simulink model "model"  (Simulink 7.7)
settings: Solver=ode45  StartTime=0.0  StopTime=10000.0  RelTol=1e-3
libraries: simeventsattributes2 x23, simeventsgenerators1 x10, simeventsrouting1 x7, simeventsserver1 x5, simeventsqueue1 x2, simeventssink1 x1, simulink x1
settings Model: Creator=flp  LastModifiedBy=flp
settings SimEventsCC: propDiagAttribOutput=1  propDiagFcnCallOutput=1  propDiagStatOutput=0

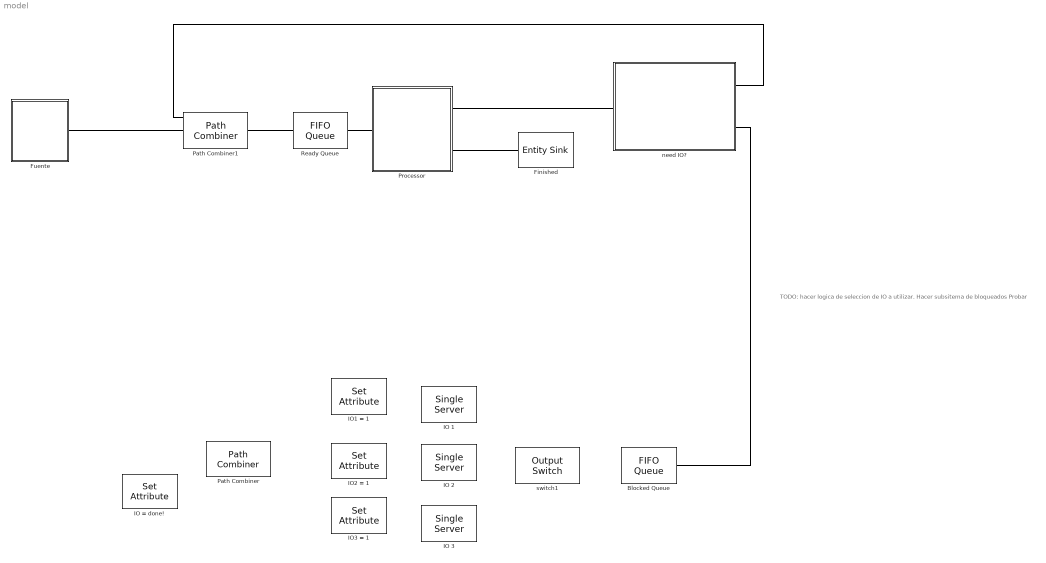
== system model ==
  note: TODO:
      |
      | hacer logica de seleccion de IO a utilizar.
      | Hacer subsitema de bloqueados
      | Probar
  Blocked Queue : simeventsqueue1/FIFO Queue  SystemSampleTime=-1  Capacity=25  EnableTOPort=off  StatNumberDeparted=Off  StatNumberInBlock=Off  StatPendingEntity=Off  StatAverageWait=Off  StatAverageQueueLength=Off  StatNumberTimedout=Off
  Finished : simeventssink1/Entity Sink  SystemSampleTime=-1  AvailableForArrivals=on  StatNumberArrived=Off
  Fuente : Subsystem
  IO 1 : simeventsserver1/Single Server  SystemSampleTime=-1  ServiceTimeFrom=Signal port t  ServiceTime=1  AttributeName=ServiceTime  PriorityServiceCompletion=500  PermitPreemption=off  SortingAttributeName=PriorityAttributeName  SortingDirection=Ascending  WriteToAttribute=off  ResidualAttributeName=ResidualServiceTime  CreateAttribute=on  EnableTOPort=off  StatNumberDeparted=Off  StatNumberInBlock=Off  StatNumberPreempted=Off  StatPendingEntity=Off  StatAverageWait=Off  StatUtilization=Off  StatNumberTimedout=Off
  IO 2 : simeventsserver1/Single Server  SystemSampleTime=-1  ServiceTimeFrom=Signal port t  ServiceTime=1  AttributeName=ServiceTime  PriorityServiceCompletion=500  PermitPreemption=off  SortingAttributeName=PriorityAttributeName  SortingDirection=Ascending  WriteToAttribute=off  ResidualAttributeName=ResidualServiceTime  CreateAttribute=on  EnableTOPort=off  StatNumberDeparted=Off  StatNumberInBlock=Off  StatNumberPreempted=Off  StatPendingEntity=Off  StatAverageWait=Off  StatUtilization=Off  StatNumberTimedout=Off
  IO 3 : simeventsserver1/Single Server  SystemSampleTime=-1  ServiceTimeFrom=Signal port t  ServiceTime=1  AttributeName=ServiceTime  PriorityServiceCompletion=500  PermitPreemption=off  SortingAttributeName=PriorityAttributeName  SortingDirection=Ascending  WriteToAttribute=off  ResidualAttributeName=ResidualServiceTime  CreateAttribute=on  EnableTOPort=off  StatNumberDeparted=Off  StatNumberInBlock=Off  StatNumberPreempted=Off  StatPendingEntity=Off  StatAverageWait=Off  StatUtilization=Off  StatNumberTimedout=Off
  IO = done! : simeventsattributes2/Set Attribute  SystemSampleTime=-1  AttributeFrom=Dialog  AttributeName=Attribute1  AttributeTreatAsVector=1  AttributeValue=1  AttributeCreate=on  StatNumberDeparted=Off  EvaluatedAttributeValue={1}
  IO1 = 1 : simeventsattributes2/Set Attribute  SystemSampleTime=-1  AttributeFrom=Signal port  AttributeName=current_process_time  AttributeTreatAsVector=1  AttributeValue=1  AttributeCreate=on  StatNumberDeparted=Off  EvaluatedAttributeValue={[]}
  IO2 = 1 : simeventsattributes2/Set Attribute  SystemSampleTime=-1  AttributeFrom=Signal port  AttributeName=current_process_time  AttributeTreatAsVector=1  AttributeValue=1  AttributeCreate=on  StatNumberDeparted=Off  EvaluatedAttributeValue={[]}
  IO3 = 1 : simeventsattributes2/Set Attribute  SystemSampleTime=-1  AttributeFrom=Signal port  AttributeName=current_process_time  AttributeTreatAsVector=1  AttributeValue=1  AttributeCreate=on  StatNumberDeparted=Off  EvaluatedAttributeValue={[]}
  Path Combiner : simeventsrouting1/Path Combiner  SystemSampleTime=-1  NumberInputPorts=3  InputPortPrecedence=IN1 port  InitialSeed=45675  SpecifyEventPriority=off  PriorityPathCombinerPortPrecedenceSelection=4100  StatNumberDeparted=Off  StatLastArrivalPort=Off  EvaluatedNumPorts=3
  Path Combiner1 : simeventsrouting1/Path Combiner  SystemSampleTime=-1  NumberInputPorts=3  InputPortPrecedence=IN1 port  InitialSeed=45675  SpecifyEventPriority=off  PriorityPathCombinerPortPrecedenceSelection=4100  StatNumberDeparted=Off  StatLastArrivalPort=Off  EvaluatedNumPorts=3
  Processor : Subsystem
  Ready Queue : simeventsqueue1/FIFO Queue  SystemSampleTime=-1  Capacity=40  EnableTOPort=off  StatNumberDeparted=Off  StatNumberInBlock=Off  StatPendingEntity=Off  StatAverageWait=Off  StatAverageQueueLength=Off  StatNumberTimedout=Off
  need IO? : Subsystem
  switch1 : simeventsrouting1/Output Switch  SystemSampleTime=-1  NumberOutputPorts=3  SwitchingCriterion=From attribute  InitialSeed=34567  AttributeName=Attribute1  InitialConditionsOpt=off  InitialConditions=1  EntityBufferOpt=off  SpecifyEventPriority=off  PriorityOutputSwitchSelectPort=4100  TimeoutPortOpt=off  StatNumberDeparted=Off  StatNumberTimedOut=Off  StatPendingEntity=Off  StatLastDeparturePort=Off  EvaluatedNumPorts=3
  connections:
  Ready Queue/RConn1 -- Processor/LConn1
  Processor/RConn2 -- Finished/LConn1
  Processor/RConn1 -- need IO?/LConn1
  Fuente/RConn1 -- Path Combiner1/LConn2
  need IO?/RConn1 -- Path Combiner1/LConn1
  Path Combiner1/RConn1 -- Ready Queue/LConn1
  need IO?/RConn2 -- Blocked Queue/LConn1

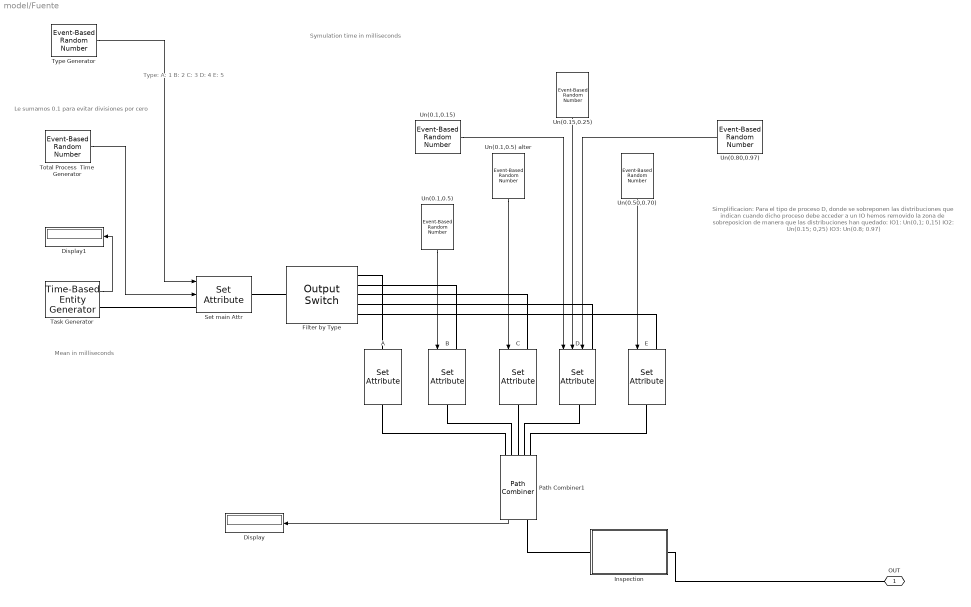
== system model/Fuente ==
  note: Type:
      |
      | A: 1
      | B: 2
      | C: 3
      | D: 4
      | E: 5
  note: Mean in milliseconds
  note: Symulation time in milliseconds
  note: Simplificacion:
      | Para el tipo de proceso D, donde se sobreponen
      | las distribuciones que indican cuando dicho proceso
      | debe acceder a un IO hemos removido la
      | zona de sobreposicion de manera que las
      | distribuciones han quedado:
      |
      | IO1: Un(0,1; 0,15)
      | IO2: Un(0.15; 0,25)
      | IO3: Un(0.8; 0.97)
  note: Le sumamos 0.1 para
      | evitar divisiones por cero
  A : simeventsattributes2/Set Attribute  SystemSampleTime=-1  AttributeFrom=Dialog|Dialog|Dialog  AttributeName=IO1|IO2|IO3  AttributeTreatAsVector=1|1|1  AttributeValue=0|0|0  AttributeCreate=on  StatNumberDeparted=Off  EvaluatedAttributeValue={0;0;0}
  B : simeventsattributes2/Set Attribute  SystemSampleTime=-1  AttributeFrom=Signal port|Dialog|Dialog  AttributeName=IO1|IO2|IO3  AttributeTreatAsVector=1|1|1  AttributeValue=1|0|0  AttributeCreate=on  StatNumberDeparted=Off  EvaluatedAttributeValue={[];0;0}
  C : simeventsattributes2/Set Attribute  SystemSampleTime=-1  AttributeFrom=Dialog|Signal port|Dialog  AttributeName=IO1|IO2|IO3  AttributeTreatAsVector=1|1|1  AttributeValue=0|1|0  AttributeCreate=on  StatNumberDeparted=Off  EvaluatedAttributeValue={0;[];0}
  D : simeventsattributes2/Set Attribute  SystemSampleTime=-1  AttributeFrom=Signal port|Signal port|Signal port  AttributeName=IO1|IO2|IO3  AttributeTreatAsVector=1|1|1  AttributeValue=1|1|1  AttributeCreate=on  StatNumberDeparted=Off  EvaluatedAttributeValue={[];[];[]}
  Display : Display
  Display1 : Display
  E : simeventsattributes2/Set Attribute  SystemSampleTime=-1  AttributeFrom=Dialog|Dialog|Signal port  AttributeName=IO1|IO2|IO3  AttributeTreatAsVector=1|1|1  AttributeValue=0|0|1  AttributeCreate=on  StatNumberDeparted=Off  EvaluatedAttributeValue={0;0;[]}
  Filter by Type : simeventsrouting1/Output Switch  SystemSampleTime=-1  NumberOutputPorts=5  SwitchingCriterion=From attribute  InitialSeed=34567  AttributeName=type  InitialConditionsOpt=off  InitialConditions=1  EntityBufferOpt=off  SpecifyEventPriority=off  PriorityOutputSwitchSelectPort=4100  TimeoutPortOpt=off  StatNumberDeparted=Off  StatNumberTimedOut=Off  StatPendingEntity=Off  StatLastDeparturePort=Off  EvaluatedNumPorts=5
  Inspection : Subsystem
  Path Combiner1 : simeventsrouting1/Path Combiner  SystemSampleTime=-1  NumberInputPorts=5  InputPortPrecedence=IN1 port  InitialSeed=45675  SpecifyEventPriority=off  PriorityPathCombinerPortPrecedenceSelection=4100  StatNumberDeparted=On  StatLastArrivalPort=Off  EvaluatedNumPorts=5
  Set main Attr : simeventsattributes2/Set Attribute  SystemSampleTime=-1  AttributeFrom=Signal port|Signal port|Dialog  AttributeName=type|total_process_time|current_process_time  AttributeTreatAsVector=1|1|1  AttributeValue=1|1|0  AttributeCreate=on  StatNumberDeparted=Off  EvaluatedAttributeValue={[];[];0}
  Task Generator : simeventsgenerators1/Entity Generators/Time-Based Entity Generator  SystemSampleTime=-1  GenerateEntitiesUpon=Intergeneration time from dialog  Distribution=Exponential  Minimum=0  Maximum=1  Mean=212.8  InitialSeed=1234  Period=1  PriorityEntityGeneration=300  GenerateEntityAtSimulationStart=on  ResponseWhenBlocked=Pause generation  ResponseWhenUnblocked=Immediate restart  EntityType=Blank  StatNumberDeparted=On  StatPendingEntity=Off  StatAverageIntergenerationTime=Off
  Total Process  Time Generator : simeventsgenerators1/Signal Generators/Event-Based Random Number  SystemSampleTime=-1  distribution=Gaussian (normal)  meanExp=1  minUnif=1  maxUnif=1  pOneBern=0.25  pSuccessBino=0.5  numTrialBino=1  meanNorm=200  stdNorm=40  minTri=1  maxTri=3  modeTri=2  thresholdLogn=0  scaleLogn=1  shapeLogn=1  pSuccessGeo=0.5  meanPoiss=1  thresholdLogl=0  scaleLogl=1  thresholdGam=0  scaleGam=1  shapeGam=1  minBeta=0  maxBeta=1  shape1Beta=1  shape2Beta=1  minUnid=0  maxUnid=1  numValueUnid=2  thresholdWbl=0  scaleWbl=1  shapeWbl=1  valueVecCont=[0 1]  cdfVecCont=[0 1]  valueVecDisc=[0 1]  probVecDisc=[0.5 0.5]  seed=12357632  IsProcessed=on  isConnected=1
  Type Generator : simeventsgenerators1/Signal Generators/Event-Based Random Number  SystemSampleTime=-1  distribution=Arbitrary discrete  meanExp=1  minUnif=1  maxUnif=1  pOneBern=0.25  pSuccessBino=0.5  numTrialBino=1  meanNorm=0  stdNorm=1  minTri=1  maxTri=3  modeTri=2  thresholdLogn=0  scaleLogn=1  shapeLogn=1  pSuccessGeo=0.5  meanPoiss=1  thresholdLogl=0  scaleLogl=1  thresholdGam=0  scaleGam=1  shapeGam=1  minBeta=0  maxBeta=1  shape1Beta=1  shape2Beta=1  minUnid=0  maxUnid=1  numValueUnid=2  thresholdWbl=0  scaleWbl=1  shapeWbl=1  valueVecCont=[0 1]  cdfVecCont=[0 1]  valueVecDisc=[1 2 3 4 5]  probVecDisc=[0.05 0.15 0.25 0.35 0.20]  seed=5533312  IsProcessed=on  isConnected=1
  Un(0.1,0.15) : simeventsgenerators1/Signal Generators/Event-Based Random Number  SystemSampleTime=-1  distribution=Uniform  meanExp=1  minUnif=0.1  maxUnif=0.15  pOneBern=0.25  pSuccessBino=0.5  numTrialBino=1  meanNorm=200  stdNorm=40  minTri=1  maxTri=3  modeTri=2  thresholdLogn=0  scaleLogn=1  shapeLogn=1  pSuccessGeo=0.5  meanPoiss=1  thresholdLogl=0  scaleLogl=1  thresholdGam=0  scaleGam=1  shapeGam=1  minBeta=0  maxBeta=1  shape1Beta=1  shape2Beta=1  minUnid=0  maxUnid=1  numValueUnid=2  thresholdWbl=0  scaleWbl=1  shapeWbl=1  valueVecCont=[0 1]  cdfVecCont=[0 1]  valueVecDisc=[0 1]  probVecDisc=[0.5 0.5]  seed=19165  IsProcessed=on  isConnected=1
  Un(0.1,0.5) : simeventsgenerators1/Signal Generators/Event-Based Random Number  SystemSampleTime=-1  distribution=Uniform  meanExp=1  minUnif=0.1  maxUnif=0.5  pOneBern=0.25  pSuccessBino=0.5  numTrialBino=1  meanNorm=200  stdNorm=40  minTri=1  maxTri=3  modeTri=2  thresholdLogn=0  scaleLogn=1  shapeLogn=1  pSuccessGeo=0.5  meanPoiss=1  thresholdLogl=0  scaleLogl=1  thresholdGam=0  scaleGam=1  shapeGam=1  minBeta=0  maxBeta=1  shape1Beta=1  shape2Beta=1  minUnid=0  maxUnid=1  numValueUnid=2  thresholdWbl=0  scaleWbl=1  shapeWbl=1  valueVecCont=[0 1]  cdfVecCont=[0 1]  valueVecDisc=[0 1]  probVecDisc=[0.5 0.5]  seed=3786546  IsProcessed=on  isConnected=1
  Un(0.1,0.5) alter : simeventsgenerators1/Signal Generators/Event-Based Random Number  SystemSampleTime=-1  distribution=Uniform  meanExp=1  minUnif=0.1  maxUnif=0.5  pOneBern=0.25  pSuccessBino=0.5  numTrialBino=1  meanNorm=200  stdNorm=40  minTri=1  maxTri=3  modeTri=2  thresholdLogn=0  scaleLogn=1  shapeLogn=1  pSuccessGeo=0.5  meanPoiss=1  thresholdLogl=0  scaleLogl=1  thresholdGam=0  scaleGam=1  shapeGam=1  minBeta=0  maxBeta=1  shape1Beta=1  shape2Beta=1  minUnid=0  maxUnid=1  numValueUnid=2  thresholdWbl=0  scaleWbl=1  shapeWbl=1  valueVecCont=[0 1]  cdfVecCont=[0 1]  valueVecDisc=[0 1]  probVecDisc=[0.5 0.5]  seed=22382  IsProcessed=on  isConnected=1
  Un(0.15,0.25) : simeventsgenerators1/Signal Generators/Event-Based Random Number  SystemSampleTime=-1  distribution=Uniform  meanExp=1  minUnif=0.15  maxUnif=0.25  pOneBern=0.25  pSuccessBino=0.5  numTrialBino=1  meanNorm=200  stdNorm=40  minTri=1  maxTri=3  modeTri=2  thresholdLogn=0  scaleLogn=1  shapeLogn=1  pSuccessGeo=0.5  meanPoiss=1  thresholdLogl=0  scaleLogl=1  thresholdGam=0  scaleGam=1  shapeGam=1  minBeta=0  maxBeta=1  shape1Beta=1  shape2Beta=1  minUnid=0  maxUnid=1  numValueUnid=2  thresholdWbl=0  scaleWbl=1  shapeWbl=1  valueVecCont=[0 1]  cdfVecCont=[0 1]  valueVecDisc=[0 1]  probVecDisc=[0.5 0.5]  seed=25599  IsProcessed=on  isConnected=1
  Un(0.50,0.70) : simeventsgenerators1/Signal Generators/Event-Based Random Number  SystemSampleTime=-1  distribution=Uniform  meanExp=1  minUnif=0.5  maxUnif=0.7  pOneBern=0.25  pSuccessBino=0.5  numTrialBino=1  meanNorm=200  stdNorm=40  minTri=1  maxTri=3  modeTri=2  thresholdLogn=0  scaleLogn=1  shapeLogn=1  pSuccessGeo=0.5  meanPoiss=1  thresholdLogl=0  scaleLogl=1  thresholdGam=0  scaleGam=1  shapeGam=1  minBeta=0  maxBeta=1  shape1Beta=1  shape2Beta=1  minUnid=0  maxUnid=1  numValueUnid=2  thresholdWbl=0  scaleWbl=1  shapeWbl=1  valueVecCont=[0 1]  cdfVecCont=[0 1]  valueVecDisc=[0 1]  probVecDisc=[0.5 0.5]  seed=28816  IsProcessed=on  isConnected=1
  Un(0.80,0.97) : simeventsgenerators1/Signal Generators/Event-Based Random Number  SystemSampleTime=-1  distribution=Uniform  meanExp=1  minUnif=0.8  maxUnif=0.97  pOneBern=0.25  pSuccessBino=0.5  numTrialBino=1  meanNorm=200  stdNorm=40  minTri=1  maxTri=3  modeTri=2  thresholdLogn=0  scaleLogn=1  shapeLogn=1  pSuccessGeo=0.5  meanPoiss=1  thresholdLogl=0  scaleLogl=1  thresholdGam=0  scaleGam=1  shapeGam=1  minBeta=0  maxBeta=1  shape1Beta=1  shape2Beta=1  minUnid=0  maxUnid=1  numValueUnid=2  thresholdWbl=0  scaleWbl=1  shapeWbl=1  valueVecCont=[0 1]  cdfVecCont=[0 1]  valueVecDisc=[0 1]  probVecDisc=[0.5 0.5]  seed=35250  IsProcessed=on  isConnected=1
  OUT : PMIOPort  Port=1  Side=Right
  wires:
  Type Generator/1 -> Set main Attr/1
  Un(0.1,0.5)/1 -> B/1
  Un(0.1,0.5) alter/1 -> C/1
  Un(0.1,0.15)/1 -> D/1
  Un(0.15,0.25)/1 -> D/2
  Un(0.80,0.97)/1 -> D/3
  Un(0.50,0.70)/1 -> E/1
  Task Generator/1 -> Display1/1
  Path Combiner1/1 -> Display/1
  Total Process  Time Generator/1 -> Set main Attr/2
  connections:
  Filter by Type/RConn1 -- A/LConn1
  Filter by Type/RConn2 -- B/LConn1
  Filter by Type/RConn3 -- C/LConn1
  Filter by Type/RConn4 -- D/LConn1
  Filter by Type/RConn5 -- E/LConn1
  Task Generator/RConn1 -- Set main Attr/LConn1
  Set main Attr/RConn1 -- Filter by Type/LConn1
  A/RConn1 -- Path Combiner1/LConn1
  B/RConn1 -- Path Combiner1/LConn2
  C/RConn1 -- Path Combiner1/LConn3
  D/RConn1 -- Path Combiner1/LConn4
  E/RConn1 -- Path Combiner1/LConn5
  Inspection/LConn1 -- Path Combiner1/RConn1
  Inspection/RConn1 -- OUT/RConn1

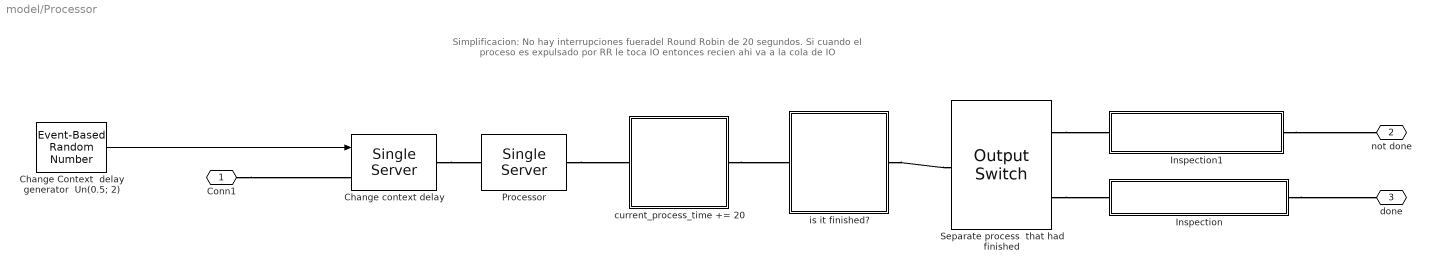
== system model/Processor ==
  note: Simplificacion:
      |
      | No hay interrupciones fueradel
      | Round Robin de 20 segundos.
      | Si cuando el proceso es expulsado por
      | RR le toca IO entonces recien ahi va a
      | la cola de IO
  Change Context  delay generator  Un(0.5; 2) : simeventsgenerators1/Signal Generators/Event-Based Random Number  SystemSampleTime=-1  distribution=Uniform  meanExp=1  minUnif=0.5  maxUnif=2  pOneBern=0.25  pSuccessBino=0.5  numTrialBino=1  meanNorm=0  stdNorm=1  minTri=1  maxTri=3  modeTri=2  thresholdLogn=0  scaleLogn=1  shapeLogn=1  pSuccessGeo=0.5  meanPoiss=1  thresholdLogl=0  scaleLogl=1  thresholdGam=0  scaleGam=1  shapeGam=1  minBeta=0  maxBeta=1  shape1Beta=1  shape2Beta=1  minUnid=0  maxUnid=1  numValueUnid=2  thresholdWbl=0  scaleWbl=1  shapeWbl=1  valueVecCont=[0 1]  cdfVecCont=[0 1]  valueVecDisc=[0 1]  probVecDisc=[0.5 0.5]  seed=55444325  IsProcessed=on  isConnected=1
  Change context delay : simeventsserver1/Single Server  SystemSampleTime=-1  ServiceTimeFrom=Signal port t  ServiceTime=1  AttributeName=ServiceTime  PriorityServiceCompletion=500  PermitPreemption=off  SortingAttributeName=PriorityAttributeName  SortingDirection=Ascending  WriteToAttribute=off  ResidualAttributeName=ResidualServiceTime  CreateAttribute=on  EnableTOPort=off  StatNumberDeparted=Off  StatNumberInBlock=Off  StatNumberPreempted=Off  StatPendingEntity=Off  StatAverageWait=Off  StatUtilization=Off  StatNumberTimedout=Off
  Inspection : Subsystem
  Inspection1 : Subsystem
  Processor : simeventsserver1/Single Server  SystemSampleTime=-1  ServiceTimeFrom=Dialog  ServiceTime=20  AttributeName=ServiceTime  PriorityServiceCompletion=500  PermitPreemption=off  SortingAttributeName=PriorityAttributeName  SortingDirection=Ascending  WriteToAttribute=off  ResidualAttributeName=ResidualServiceTime  CreateAttribute=on  EnableTOPort=off  StatNumberDeparted=Off  StatNumberInBlock=Off  StatNumberPreempted=Off  StatPendingEntity=Off  StatAverageWait=Off  StatUtilization=Off  StatNumberTimedout=Off
  Separate process  that had finished : simeventsrouting1/Output Switch  SystemSampleTime=-1  NumberOutputPorts=2  SwitchingCriterion=From attribute  InitialSeed=34567  AttributeName=done  InitialConditionsOpt=off  InitialConditions=1  EntityBufferOpt=off  SpecifyEventPriority=off  PriorityOutputSwitchSelectPort=4100  TimeoutPortOpt=off  StatNumberDeparted=Off  StatNumberTimedOut=Off  StatPendingEntity=Off  StatLastDeparturePort=Off  EvaluatedNumPorts=2
  current_process_time += 20 : Subsystem
  is it finished? : Subsystem
  Conn1 : PMIOPort  Port=1  Side=Left
  not done : PMIOPort  Port=2  Side=Right
  done : PMIOPort  Port=3  Side=Right
  wires:
  Change Context  delay generator  Un(0.5; 2)/1 -> Change context delay/1
  connections:
  Change context delay/RConn1 -- Processor/LConn1
  Processor/RConn1 -- current_process_time += 20/LConn1
  current_process_time += 20/RConn1 -- is it finished?/LConn1
  Conn1/RConn1 -- Change context delay/LConn1
  is it finished?/RConn1 -- Separate process  that had finished/LConn1
  Separate process  that had finished/RConn1 -- Inspection1/LConn1
  Separate process  that had finished/RConn2 -- Inspection/LConn1
  Inspection/RConn1 -- done/RConn1
  Inspection1/RConn1 -- not done/RConn1

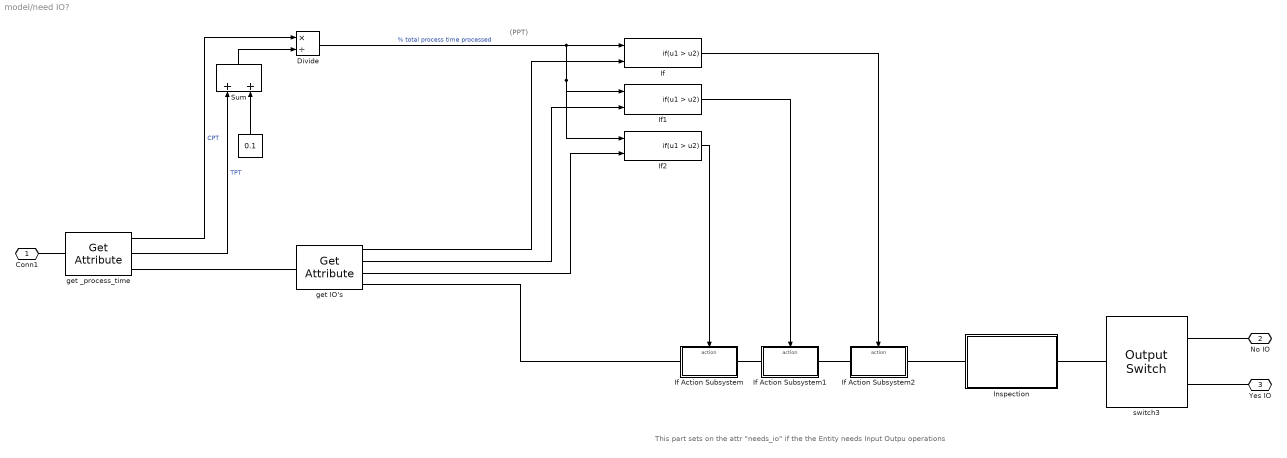
== system model/need IO? ==
  note: (PPT)
  note: This part sets on the attr "needs_io" if the the Entity needs Input Outpu operations
  "   " : Constant  Value=0.1
  Divide : Product  Inputs=*/
  If : If  NumInputs=2  IfExpression=u1 > u2  ShowElse=off
  If Action Subsystem : Subsystem  TreatAsAtomicUnit=on
  If Action Subsystem1 : Subsystem  TreatAsAtomicUnit=on
  If Action Subsystem2 : Subsystem  TreatAsAtomicUnit=on
  If1 : If  NumInputs=2  IfExpression=u1 > u2  ShowElse=off
  If2 : If  NumInputs=2  IfExpression=u1 > u2  ShowElse=off
  Inspection : Subsystem
  Sum : Sum
  get IO's : simeventsattributes2/Get Attribute  SystemSampleTime=-1  AttributeName=IO1|IO2|IO3  AttributeMissing=Error|Error|Error  AttributeDefaultValue=1|1|1  AttributeSendTiming=After entity departure|After entity departure|After entity departure  AttributeTreatAsVector=1|1|1  StatNumberDeparted=Off  EvaluatedDefaultAttributeValue={[];[];[]}
  get _process_time : simeventsattributes2/Get Attribute  SystemSampleTime=-1  AttributeName=current_process_time|total_process_time  AttributeMissing=Error|Error  AttributeDefaultValue=1|1  AttributeSendTiming=After entity departure|After entity departure  AttributeTreatAsVector=1|1  StatNumberDeparted=Off  EvaluatedDefaultAttributeValue={[];[]}
  switch3 : simeventsrouting1/Output Switch  SystemSampleTime=-1  NumberOutputPorts=2  SwitchingCriterion=From attribute  InitialSeed=34567  AttributeName=needs_io  InitialConditionsOpt=off  InitialConditions=1  EntityBufferOpt=off  SpecifyEventPriority=off  PriorityOutputSwitchSelectPort=4100  TimeoutPortOpt=off  StatNumberDeparted=Off  StatNumberTimedOut=Off  StatPendingEntity=Off  StatLastDeparturePort=Off  EvaluatedNumPorts=2
  Conn1 : PMIOPort  Port=1  Side=Left
  No IO : PMIOPort  Port=2  Side=Right
  Yes IO : PMIOPort  Port=3  Side=Right
  wires:
  get _process_time/1 -> Divide/1  "CPT"
  get _process_time/2 -> Sum/1  "TPT"
  Divide/1 -> If/1, If2/1, If1/1  "% total process time processed"
  Sum/1 -> Divide/2
  "   "/1 -> Sum/2
  get IO's/1 -> If/2
  get IO's/2 -> If1/2
  get IO's/3 -> If2/2
  If1/1 -> If Action Subsystem1/Action
  If2/1 -> If Action Subsystem/Action
  If/1 -> If Action Subsystem2/Action
  connections:
  get _process_time/RConn1 -- get IO's/LConn1
  Conn1/RConn1 -- get _process_time/LConn1
  No IO/RConn1 -- switch3/RConn1
  Yes IO/RConn1 -- switch3/RConn2
  If Action Subsystem/RConn1 -- If Action Subsystem1/LConn1
  If Action Subsystem1/RConn1 -- If Action Subsystem2/LConn1
  get IO's/RConn1 -- If Action Subsystem/LConn1
  Inspection/RConn1 -- switch3/LConn1
  If Action Subsystem2/RConn1 -- Inspection/LConn1

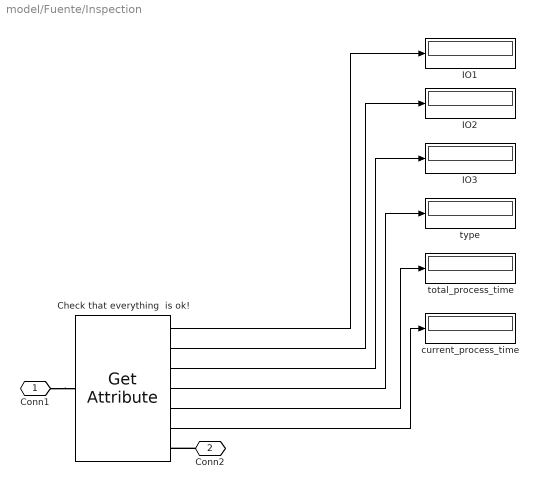
== system model/Fuente/Inspection ==
  Check that everything  is ok! : simeventsattributes2/Get Attribute  SystemSampleTime=-1  AttributeName=IO1|IO2|IO3|type|total_process_time|current_process_time  AttributeMissing=Error|Error|Error|Error|Error|Error  AttributeDefaultValue=1|1|1|1|1|1  AttributeSendTiming=After entity departure|After entity departure|After entity departure|After entity departure|After entity departure|After entity departure  AttributeTreatAsVector=1|1|1|1|1|1  StatNumberDeparted=Off  EvaluatedDefaultAttributeValue={[];[];[];[];[];[]}
  IO1 : Display
  IO2 : Display
  IO3 : Display
  current_process_time : Display
  total_process_time : Display
  type : Display
  Conn1 : PMIOPort  Port=1  Side=Left
  Conn2 : PMIOPort  Port=2  Side=Right
  wires:
  Check that everything  is ok!/1 -> IO1/1
  Check that everything  is ok!/2 -> IO2/1
  Check that everything  is ok!/3 -> IO3/1
  Check that everything  is ok!/4 -> type/1
  Check that everything  is ok!/5 -> total_process_time/1
  Check that everything  is ok!/6 -> current_process_time/1
  connections:
  Conn1/RConn1 -- Check that everything  is ok!/LConn1
  Conn2/RConn1 -- Check that everything  is ok!/RConn1

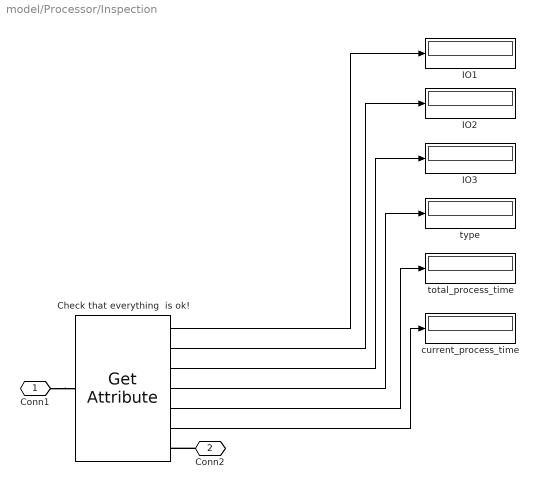
== system model/Processor/Inspection ==
  Check that everything  is ok! : simeventsattributes2/Get Attribute  SystemSampleTime=-1  AttributeName=IO1|IO2|IO3|type|total_process_time|current_process_time  AttributeMissing=Error|Error|Error|Error|Error|Error  AttributeDefaultValue=1|1|1|1|1|1  AttributeSendTiming=After entity departure|After entity departure|After entity departure|After entity departure|After entity departure|After entity departure  AttributeTreatAsVector=1|1|1|1|1|1  StatNumberDeparted=Off  EvaluatedDefaultAttributeValue={[];[];[];[];[];[]}
  IO1 : Display
  IO2 : Display
  IO3 : Display
  current_process_time : Display
  total_process_time : Display
  type : Display
  Conn1 : PMIOPort  Port=1  Side=Left
  Conn2 : PMIOPort  Port=2  Side=Right
  wires:
  Check that everything  is ok!/1 -> IO1/1
  Check that everything  is ok!/2 -> IO2/1
  Check that everything  is ok!/3 -> IO3/1
  Check that everything  is ok!/4 -> type/1
  Check that everything  is ok!/5 -> total_process_time/1
  Check that everything  is ok!/6 -> current_process_time/1
  connections:
  Conn1/RConn1 -- Check that everything  is ok!/LConn1
  Conn2/RConn1 -- Check that everything  is ok!/RConn1

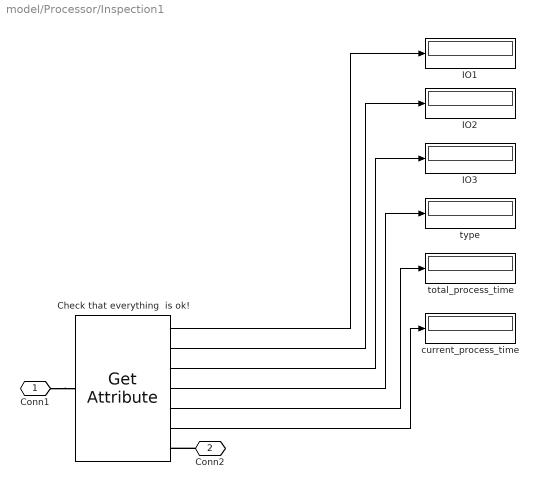
== system model/Processor/Inspection1 ==
  Check that everything  is ok! : simeventsattributes2/Get Attribute  SystemSampleTime=-1  AttributeName=IO1|IO2|IO3|type|total_process_time|current_process_time  AttributeMissing=Error|Error|Error|Error|Error|Error  AttributeDefaultValue=1|1|1|1|1|1  AttributeSendTiming=After entity departure|After entity departure|After entity departure|After entity departure|After entity departure|After entity departure  AttributeTreatAsVector=1|1|1|1|1|1  StatNumberDeparted=Off  EvaluatedDefaultAttributeValue={[];[];[];[];[];[]}
  IO1 : Display
  IO2 : Display
  IO3 : Display
  current_process_time : Display
  total_process_time : Display
  type : Display
  Conn1 : PMIOPort  Port=1  Side=Left
  Conn2 : PMIOPort  Port=2  Side=Right
  wires:
  Check that everything  is ok!/1 -> IO1/1
  Check that everything  is ok!/2 -> IO2/1
  Check that everything  is ok!/3 -> IO3/1
  Check that everything  is ok!/4 -> type/1
  Check that everything  is ok!/5 -> total_process_time/1
  Check that everything  is ok!/6 -> current_process_time/1
  connections:
  Conn1/RConn1 -- Check that everything  is ok!/LConn1
  Conn2/RConn1 -- Check that everything  is ok!/RConn1

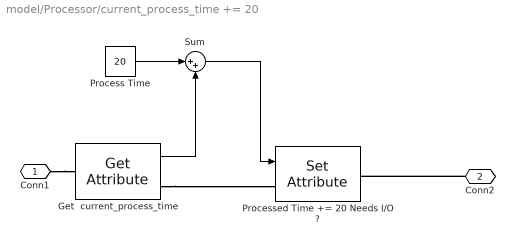
== system model/Processor/current_process_time += 20 ==
  Get  current_process_time : simeventsattributes2/Get Attribute  SystemSampleTime=-1  AttributeName=current_process_time  AttributeMissing=Error  AttributeDefaultValue=1  AttributeSendTiming=After entity departure  AttributeTreatAsVector=1  StatNumberDeparted=Off  EvaluatedDefaultAttributeValue={[]}
  Process Time : Constant  Value=20
  Processed Time += 20 Needs I/O ? : simeventsattributes2/Set Attribute  SystemSampleTime=-1  AttributeFrom=Signal port  AttributeName=current_process_time  AttributeTreatAsVector=1  AttributeValue=1  AttributeCreate=on  StatNumberDeparted=Off  EvaluatedAttributeValue={[]}
  Sum : Sum  Inputs=|++
  Conn1 : PMIOPort  Port=1  Side=Left
  Conn2 : PMIOPort  Port=2  Side=Right
  wires:
  Get  current_process_time/1 -> Sum/2
  Sum/1 -> Processed Time += 20 Needs I/O ?/1
  Process Time/1 -> Sum/1
  connections:
  Get  current_process_time/RConn1 -- Processed Time += 20 Needs I/O ?/LConn1
  Conn1/RConn1 -- Get  current_process_time/LConn1
  Conn2/RConn1 -- Processed Time += 20 Needs I/O ?/RConn1

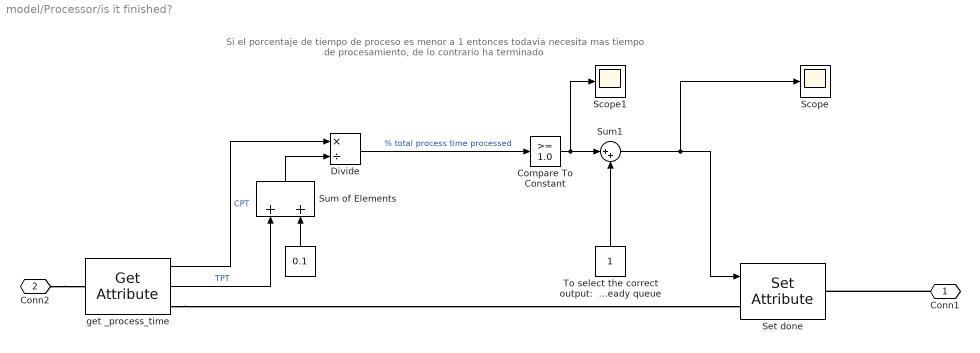
== system model/Processor/is it finished? ==
  note: Si el porcentaje de tiempo de proceso es menor a 1
      | entonces todavia necesita mas tiempo de procesamiento,
      | de lo contrario ha terminado
  "   " : Constant  Value=0.1
  Compare To Constant : simulink/Logic and Bit Operations/Compare To Constant  SystemSampleTime=-1  relop=>=  const=1.0  LogicOutDataTypeMode=uint8
  Divide : Product  Inputs=*/
  Scope : Scope
  Scope1 : Scope
  Set done : simeventsattributes2/Set Attribute  SystemSampleTime=-1  AttributeFrom=Signal port  AttributeName=done  AttributeTreatAsVector=1  AttributeValue=1  AttributeCreate=on  StatNumberDeparted=Off  EvaluatedAttributeValue={[]}
  Sum of Elements : Sum
  Sum1 : Sum  Inputs=|++
  To select the correct output:  finished or ready queue : Constant
  get _process_time : simeventsattributes2/Get Attribute  SystemSampleTime=-1  AttributeName=current_process_time|total_process_time  AttributeMissing=Error|Error  AttributeDefaultValue=1|1  AttributeSendTiming=After entity departure|After entity departure  AttributeTreatAsVector=1|1  StatNumberDeparted=Off  EvaluatedDefaultAttributeValue={[];[]}
  Conn1 : PMIOPort  Port=1  Side=Right
  Conn2 : PMIOPort  Port=2  Side=Left
  wires:
  get _process_time/1 -> Divide/1  "CPT"
  get _process_time/2 -> Sum of Elements/1  "TPT"
  Sum1/1 -> Set done/1, Scope/1
  Divide/1 -> Compare To Constant/1  "% total process time processed"
  Compare To Constant/1 -> Sum1/1, Scope1/1
  To select the correct output:  finished or ready queue/1 -> Sum1/2
  Sum of Elements/1 -> Divide/2
  "   "/1 -> Sum of Elements/2
  connections:
  get _process_time/RConn1 -- Set done/LConn1
  Conn1/RConn1 -- Set done/RConn1
  Conn2/RConn1 -- get _process_time/LConn1

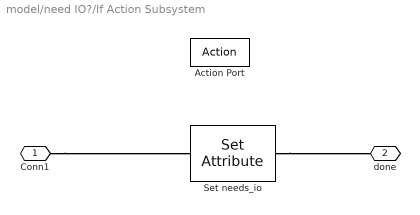
== system model/need IO?/If Action Subsystem ==
  Action Port : ActionPort  ActionType=then
  Set needs_io : simeventsattributes2/Set Attribute  SystemSampleTime=-1  AttributeFrom=Dialog  AttributeName=needs_io  AttributeTreatAsVector=1  AttributeValue=2  AttributeCreate=on  StatNumberDeparted=Off  EvaluatedAttributeValue={2}
  Conn1 : PMIOPort  Port=1  Side=Left
  done : PMIOPort  Port=2  Side=Right
  connections:
  Conn1/RConn1 -- Set needs_io/LConn1
  Set needs_io/RConn1 -- done/RConn1

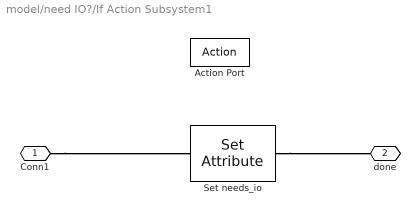
== system model/need IO?/If Action Subsystem1 ==
  Action Port : ActionPort  ActionType=then
  Set needs_io : simeventsattributes2/Set Attribute  SystemSampleTime=-1  AttributeFrom=Dialog  AttributeName=needs_io  AttributeTreatAsVector=1  AttributeValue=2  AttributeCreate=on  StatNumberDeparted=Off  EvaluatedAttributeValue={2}
  Conn1 : PMIOPort  Port=1  Side=Left
  done : PMIOPort  Port=2  Side=Right
  connections:
  Conn1/RConn1 -- Set needs_io/LConn1
  Set needs_io/RConn1 -- done/RConn1

== system model/need IO?/If Action Subsystem2 ==
  Action Port : ActionPort  ActionType=then
  Set needs_io : simeventsattributes2/Set Attribute  SystemSampleTime=-1  AttributeFrom=Dialog  AttributeName=needs_io  AttributeTreatAsVector=1  AttributeValue=2  AttributeCreate=on  StatNumberDeparted=Off  EvaluatedAttributeValue={2}
  Conn1 : PMIOPort  Port=1  Side=Left
  done : PMIOPort  Port=2  Side=Right
  connections:
  Conn1/RConn1 -- Set needs_io/LConn1
  Set needs_io/RConn1 -- done/RConn1

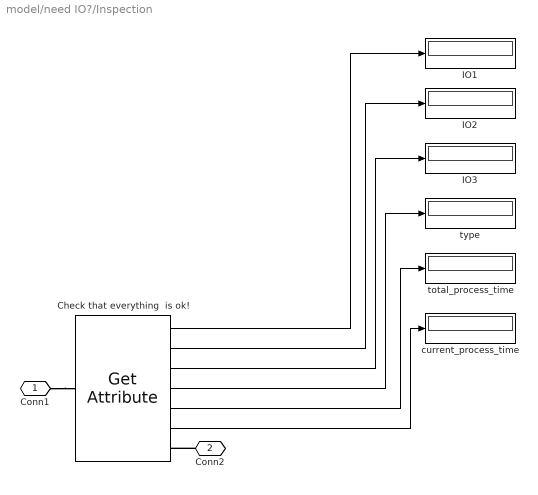
== system model/need IO?/Inspection ==
  Check that everything  is ok! : simeventsattributes2/Get Attribute  SystemSampleTime=-1  AttributeName=IO1|IO2|IO3|type|total_process_time|current_process_time  AttributeMissing=Error|Error|Error|Error|Error|Error  AttributeDefaultValue=1|1|1|1|1|1  AttributeSendTiming=After entity departure|After entity departure|After entity departure|After entity departure|After entity departure|After entity departure  AttributeTreatAsVector=1|1|1|1|1|1  StatNumberDeparted=Off  EvaluatedDefaultAttributeValue={[];[];[];[];[];[]}
  IO1 : Display
  IO2 : Display
  IO3 : Display
  current_process_time : Display
  total_process_time : Display
  type : Display
  Conn1 : PMIOPort  Port=1  Side=Left
  Conn2 : PMIOPort  Port=2  Side=Right
  wires:
  Check that everything  is ok!/1 -> IO1/1
  Check that everything  is ok!/2 -> IO2/1
  Check that everything  is ok!/3 -> IO3/1
  Check that everything  is ok!/4 -> type/1
  Check that everything  is ok!/5 -> total_process_time/1
  Check that everything  is ok!/6 -> current_process_time/1
  connections:
  Conn1/RConn1 -- Check that everything  is ok!/LConn1
  Conn2/RConn1 -- Check that everything  is ok!/RConn1
